simulink model "GravSimple"  (R2020b)
settings: Solver=VariableStepAuto  StartTime=0.0  StopTime=20  MaxStep=0.001  RelTol=1e-3
values from neighbouring files (symbols this model uses):
  b = 1e4    (= 10000)    [calcGrav.m]
  Fpin0 = 4*k0*tauM0/2/(g*1000)    [calcGrav.m]
  GBr = 39.9    [calcGrav.m]
  K = nc*(EA./Ds)    [calcGrav.m]
  M1 = alfa*mc + Mmot + Mwin + Msh    (= 57445.7643225)    [calcGrav.m]
  M2 = (1-alfa)*mc + M    (= 50290)    [calcGrav.m]
  rw0 = 0.562/2    (= 0.281)    [calcGrav.m]
  tau_em = 60e-3    (= 0.06)    [calcGrav.m]    (also in main.m)
  tau_m = tau_w/GB.r    [main.m]
  tau_max = tauM0    [calcGrav.m]
  tauM0 = (M + mc)*g/4/k0    [calcGrav.m]
undefined symbols (not defined in the file or in its folder): PID
libraries: cstblocks x1, pid_lib x1
settings Model: Creator=Pawel  LastModifiedBy=Pawel

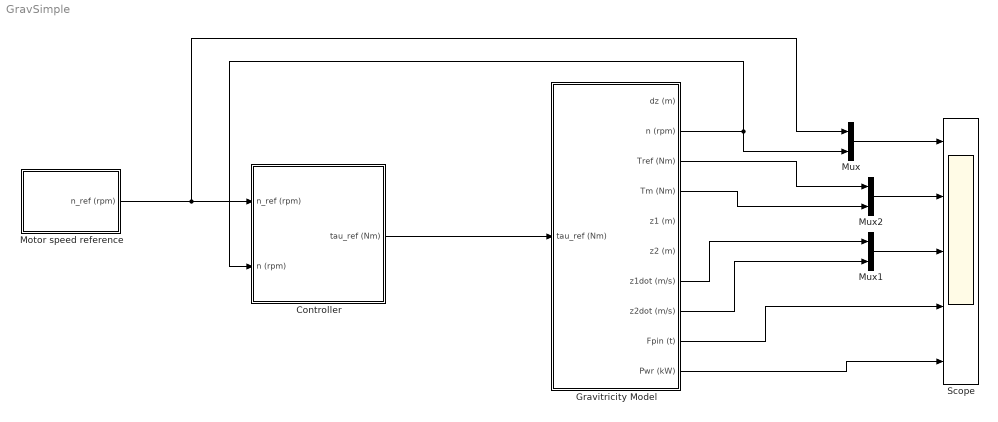
== system GravSimple ==
  Controller : Subsystem
  Gravitricity Model : Subsystem
  Motor speed reference : Subsystem
  Mux : Mux  Inputs=2
  Mux1 : Mux  Inputs=2
  Mux2 : Mux  Inputs=2
  Scope : Scope  NumInputPorts=5
  wires:
  Motor speed reference/1(n_ref (rpm)) -> Mux/1, Controller/1(n_ref (rpm))
  Gravitricity Model/2(n (rpm)) -> Mux/2, Controller/2(n (rpm))
  Controller/1(tau_ref (Nm)) -> Gravitricity Model/1(tau_ref (Nm))
  Mux/1 -> Scope/1
  Gravitricity Model/10(Pwr (kW)) -> Scope/5
  Mux1/1 -> Scope/3
  Gravitricity Model/9(Fpin (t)) -> Scope/4
  Gravitricity Model/7(z1dot (m/s)) -> Mux1/1
  Gravitricity Model/8(z2dot (m/s)) -> Mux1/2
  Mux2/1 -> Scope/2
  Gravitricity Model/3(Tref (Nm)) -> Mux2/1
  Gravitricity Model/4(Tm (Nm)) -> Mux2/2

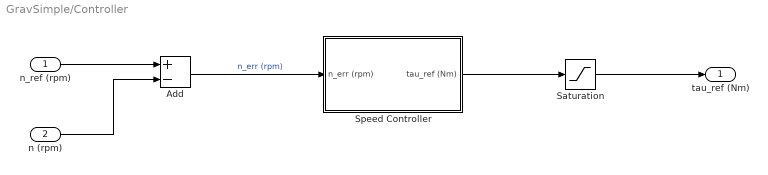
== system GravSimple/Controller ==
  n_ref (rpm) : Inport
  n (rpm) : Inport  Port=2
  Add : Sum  Inputs=+-
  Saturation : Saturate  UpperLimit=tau_max  LowerLimit=-tau_max
  Speed Controller : Subsystem  Variant=on  VariantControlMode=label  LabelModeActiveChoice=Speed_Ctrl_OL
  tau_ref (Nm) : Outport
  wires:
  n_ref (rpm)/1 -> Add/1
  n (rpm)/1 -> Add/2
  Add/1 -> Speed Controller/1(n_err (rpm))  "n_err (rpm)"
  Speed Controller/1(tau_ref (Nm)) -> Saturation/1
  Saturation/1 -> tau_ref (Nm)/1

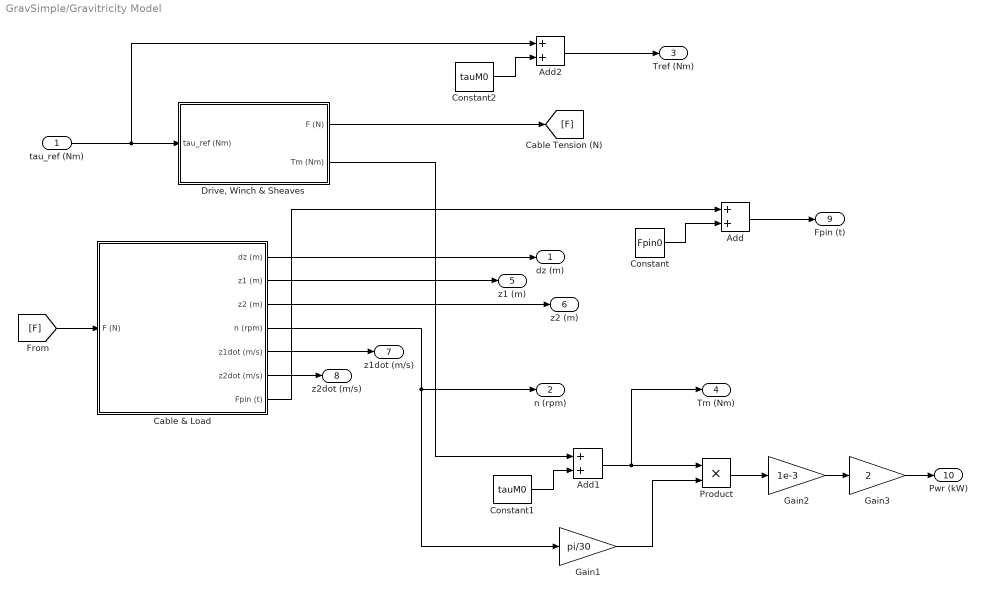
== system GravSimple/Gravitricity Model ==
  tau_ref (Nm) : Inport
  Add : Sum
  Add1 : Sum
  Add2 : Sum
  Cable & Load : Subsystem  Variant=on  VariantControlMode=label  LabelModeActiveChoice=Load_2
  Constant : Constant  Value=Fpin0
  Constant1 : Constant  Value=tauM0
  Constant2 : Constant  Value=tauM0
  "Drive, Winch & Sheaves" : Subsystem  Variant=on  VariantControlMode=label  LabelModeActiveChoice=Drive_2
  Gain1 : Gain  Gain=pi/30
  Gain2 : Gain  Gain=1e-3
  Gain3 : Gain  Gain=2
  Product : Product
  dz (m) : Outport
  n (rpm) : Outport  Port=2
  Tref (Nm) : Outport  Port=3
  Tm (Nm) : Outport  Port=4
  z1 (m) : Outport  Port=5
  z2 (m) : Outport  Port=6
  z1dot (m/s) : Outport  Port=7
  z2dot (m/s) : Outport  Port=8
  Fpin (t) : Outport  Port=9
  Pwr (kW) : Outport  Port=10
  wires:
  tau_ref (Nm)/1 -> Add2/1, "Drive, Winch & Sheaves"/1(tau_ref (Nm))
  "Drive, Winch & Sheaves"/1(F (N)) -> [F]
  [F] -> Cable & Load/1(F (N))
  Cable & Load/1(dz (m)) -> dz (m)/1
  Cable & Load/2(z1 (m)) -> z1 (m)/1
  Cable & Load/3(z2 (m)) -> z2 (m)/1
  Cable & Load/4(n (rpm)) -> Gain1/1, n (rpm)/1
  "Drive, Winch & Sheaves"/2(Tm (Nm)) -> Add1/1
  Cable & Load/7(Fpin (t)) -> Add/1
  Add/1 -> Fpin (t)/1
  Constant/1 -> Add/2
  Constant1/1 -> Add1/2
  Add1/1 -> Tm (Nm)/1, Product/1
  Gain1/1 -> Product/2
  Product/1 -> Gain2/1
  Gain2/1 -> Gain3/1
  Constant2/1 -> Add2/2
  Add2/1 -> Tref (Nm)/1
  Cable & Load/5(z1dot (m/s)) -> z1dot (m/s)/1
  Cable & Load/6(z2dot (m/s)) -> z2dot (m/s)/1
  Gain3/1 -> Pwr (kW)/1

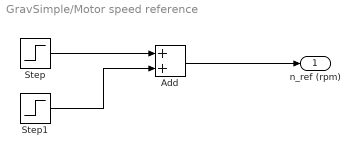
== system GravSimple/Motor speed reference ==
  Add : Sum
  Step : Step  After=1000  SampleTime=0
  Step1 : Step  Time=10  After=-1000  SampleTime=0
  n_ref (rpm) : Outport
  wires:
  Step/1 -> Add/1
  Step1/1 -> Add/2
  Add/1 -> n_ref (rpm)/1

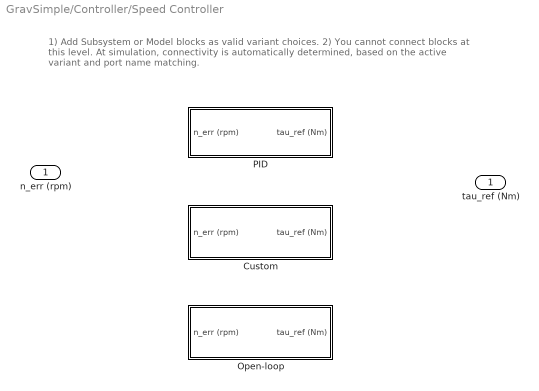
== system GravSimple/Controller/Speed Controller ==
  note: 1) Add Subsystem or Model blocks as valid variant choices.
      | 2) You cannot connect blocks at this level. At simulation, connectivity is automatically
      | determined, based on the active variant and port name matching.
  n_err (rpm) : Inport
  Custom : Subsystem  VariantControl=Speed_Ctrl_Custom
  Open-loop : Subsystem  VariantControl=Speed_Ctrl_OL
  PID : Subsystem  VariantControl=Speed_Ctrl_PID
  tau_ref (Nm) : Outport

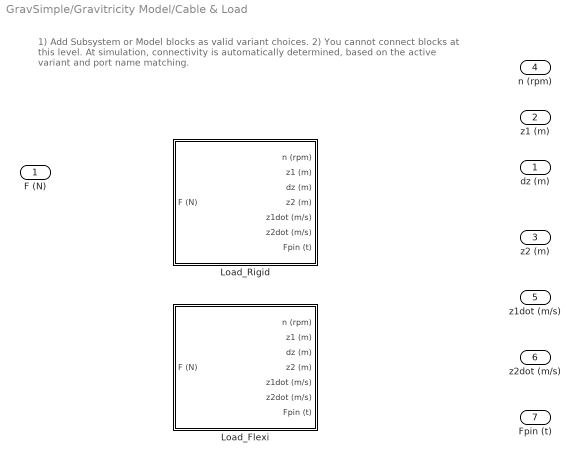
== system GravSimple/Gravitricity Model/Cable & Load ==
  note: 1) Add Subsystem or Model blocks as valid variant choices.
      | 2) You cannot connect blocks at this level. At simulation, connectivity is automatically
      | determined, based on the active variant and port name matching.
  F (N) : Inport
  Load_Flexi : Subsystem  VariantControl=Load_2
  Load_Rigid : Subsystem  VariantControl=Load_1
  dz (m) : Outport
  z1 (m) : Outport  Port=2
  z2 (m) : Outport  Port=3
  n (rpm) : Outport  Port=4
  z1dot (m/s) : Outport  Port=5
  z2dot (m/s) : Outport  Port=6
  Fpin (t) : Outport  Port=7

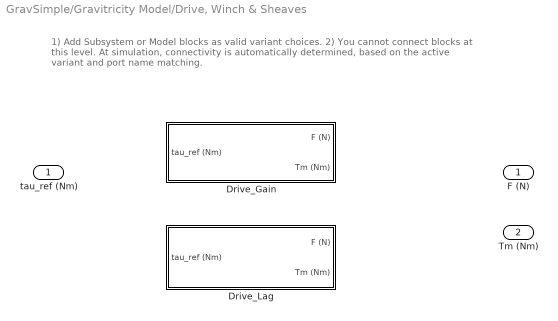
== system GravSimple/Gravitricity Model/Drive, Winch & Sheaves ==
  note: 1) Add Subsystem or Model blocks as valid variant choices.
      | 2) You cannot connect blocks at this level. At simulation, connectivity is automatically
      | determined, based on the active variant and port name matching.
  tau_ref (Nm) : Inport
  Drive_Gain : Subsystem  VariantControl=Drive_1
  Drive_Lag : Subsystem  VariantControl=Drive_2
  F (N) : Outport
  Tm (Nm) : Outport  Port=2

== system GravSimple/Controller/Speed Controller/Custom ==
  n_err (rpm) : Inport
  LTI System : cstblocks/LTI System  sys=sysC  IC=[]
  tau_ref (Nm) : Outport
  wires:
  n_err (rpm)/1 -> LTI System/1
  LTI System/1 -> tau_ref (Nm)/1

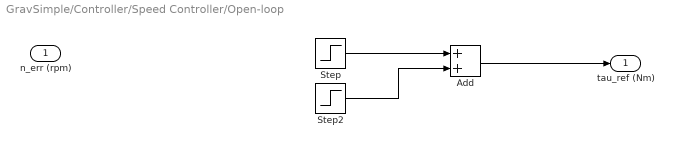
== system GravSimple/Controller/Speed Controller/Open-loop ==
  n_err (rpm) : Inport
  Add : Sum
  Step : Step  Time=5  After=0.5*tau_m  SampleTime=0
  Step2 : Step  Time=5.2  After=-0.5*tau_m  SampleTime=0
  tau_ref (Nm) : Outport
  wires:
  Add/1 -> tau_ref (Nm)/1
  Step/1 -> Add/1
  Step2/1 -> Add/2

== system GravSimple/Controller/Speed Controller/PID ==
  n_err (rpm) : Inport
  PID Controller : pid_lib/PID Controller  Controller=PID  Form=Parallel  TimeDomain=Continuous-time  UseExternalTs=off  SampleTime=-1  IntegratorMethod=Forward Euler  FilterMethod=Forward Euler  ControllerParametersSource=internal  P=PID.P  I=PID.I  D=PID.D  UseFilter=on  N=100  TunerSelectOption=Transfer Function Based (PID Tuner App)  InitialConditionSource=internal  InitialConditionForIntegrator=0  InitialConditionForFilter=0  DifferentiatorICPrevScaledInput=0  ExternalReset=none  TrackingMode=off  Kt=1  LimitOutput=off  SatLimitsSource=internal  UpperSaturationLimit=inf  LowerSaturationLimit=-inf  LinearizeAsGain=on  AntiWindupMode=none  Kb=1  POutMin=[]  POutMax=[]  IOutMin=[]  IOutMax=[]  DOutMin=[]  DOutMax=[]  NOutMin=[]  NOutMax=[]  SumOutMin=[]  SumOutMax=[]  SaturationOutMin=[]  SaturationOutMax=[]  PParamMin=[]  PParamMax=[]  IParamMin=[]  IParamMax=[]  DParamMin=[]  DParamMax=[]  NParamMin=[]  NParamMax=[]  KbParamMin=[]  KbParamMax=[]  KtParamMin=[]  KtParamMax=[]  KbOutMin=[]  KbOutMax=[]  KtOutMin=[]  KtOutMax=[]  IntegratorOutMin=[]  IntegratorOutMax=[]  FilterOutMin=[]  FilterOutMax=[]  SumI1OutMin=[]  SumI1OutMax=[]  SumI2OutMin=[]  SumI2OutMax=[]  SumI3OutMin=[]  SumI3OutMax=[]  SumI4OutMin=[]  SumI4OutMax=[]  SumDOutMin=[]  SumDOutMax=[]  DifferentiatorOutMin=[]  DifferentiatorOutMax=[]  FilterDiffOutCoefMin=[]  FilterDiffOutCoefMax=[]  ReciprocalOutMin=[]  ReciprocalOutMax=[]  SumDenOutMin=[]  SumDenOutMax=[]  SumNumOutMin=[]  SumNumOutMax=[]  DivideOutMin=[]  DivideOutMax=[]  UdiffTsProdOutMin=[]  UdiffTsProdOutMax=[]  NTsProdOutMin=[]  NTsProdOutMax=[]  UintegralTsProdOutMin=[]  UintegralTsProdOutMax=[]  UngainTsProdOutMin=[]  UngainTsProdOutMax=[]  IntegratorContinuousStateAttributes=''  IntegratorStateMustResolveToSignalObject=off  IntegratorRTWStateStorageClass=Auto  FilterContinuousStateAttributes=''  FilterStateMustResolveToSignalObject=off  FilterRTWStateStorageClass=Auto  ParallelPVariant=InternalParameters  IdealPVariant=Disabled  IVariant=InternalParameters  DVariant=InternalParameters  IntegratorVariant=Continuous  SatVariant=Disabled  AWVariant=Passthrough  PCopyVariant=Disabled  TRVariant=Disabled  FdbkBlocksVariant=Forward  IdealPFdbkVariant=Disabled  SatFdbkVariant=Disabled  DerivativeFilterVariant=ContFilter  NVariant=InternalParameters  NCopyVariant=Disabled  FilterICVariant=InternalICsFilter  IntegratorICVariant=InternalICs  ExternalResetVariant=Disabled  TRSumVariant=Passthrough  SumFdbkVariant=Disabled  SumVariant=Sum_PID  TsampFilterVariant=InternalTs  TsampNgainVariant=Passthrough  TsampIntegralVariant=Passthrough  ExternalSaturationOutDataTypeStr=Inherit: Same as second input
  tau_ref (Nm) : Outport
  wires:
  n_err (rpm)/1 -> PID Controller/1
  PID Controller/1 -> tau_ref (Nm)/1

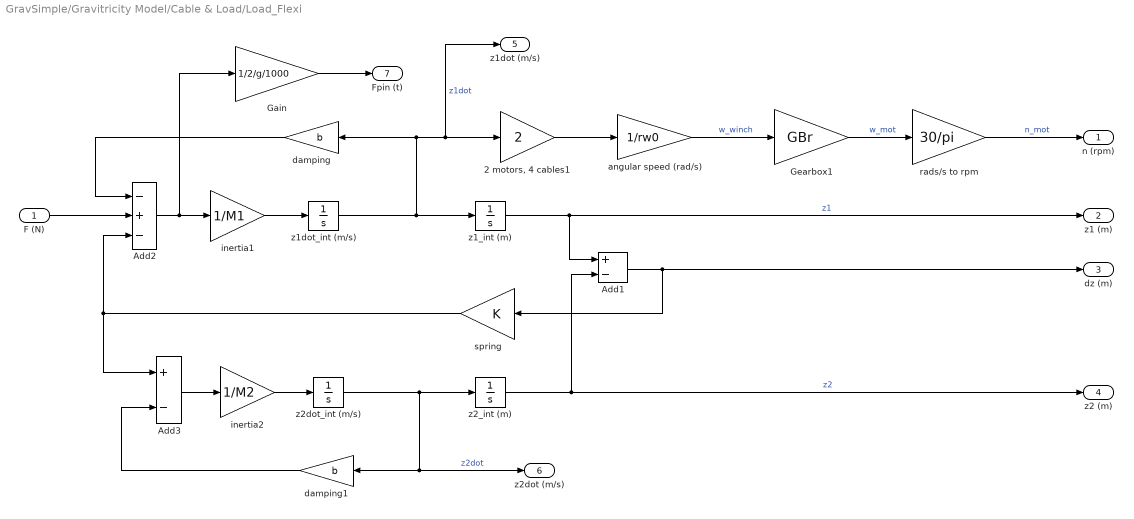
== system GravSimple/Gravitricity Model/Cable & Load/Load_Flexi ==
  F (N) : Inport
  "2 motors, 4 cables1" : Gain  Gain=2
  Add1 : Sum  Inputs=+-
  Add2 : Sum  Inputs=-+-
  Add3 : Sum  Inputs=+-
  Gain : Gain  Gain=1/2/g/1000
  Gearbox1 : Gain  Gain=GBr
  angular speed (rad/s) : Gain  Gain=1/rw0
  damping : Gain  Gain=b
  damping1 : Gain  Gain=b
  inertia1 : Gain  Gain=1/M1
  inertia2 : Gain  Gain=1/M2
  rads/s to rpm : Gain  Gain=30/pi
  spring : Gain  Gain=K
  z1_int (m) : Integrator
  z1dot_int (m/s) : Integrator
  z2_int (m) : Integrator
  z2dot_int (m/s) : Integrator
  n (rpm) : Outport
  z1 (m) : Outport  Port=2
  dz (m) : Outport  Port=3
  z2 (m) : Outport  Port=4
  z1dot (m/s) : Outport  Port=5
  z2dot (m/s) : Outport  Port=6
  Fpin (t) : Outport  Port=7
  wires:
  F (N)/1 -> Add2/2
  inertia2/1 -> z2dot_int (m/s)/1
  Add2/1 -> Gain/1, inertia1/1
  z2_int (m)/1 -> Add1/2, z2 (m)/1  "z2"
  Gearbox1/1 -> rads/s to rpm/1  "w_mot"
  angular speed (rad/s)/1 -> Gearbox1/1  "w_winch"
  z2dot_int (m/s)/1 -> z2_int (m)/1, z2dot (m/s)/1, damping1/1  "z2dot"
  inertia1/1 -> z1dot_int (m/s)/1
  z1_int (m)/1 -> Add1/1, z1 (m)/1  "z1"
  damping1/1 -> Add3/2
  Add3/1 -> inertia2/1
  z1dot_int (m/s)/1 -> z1_int (m)/1, damping/1, z1dot (m/s)/1, "2 motors, 4 cables1"/1  "z1dot"
  Add1/1 -> spring/1, dz (m)/1
  "2 motors, 4 cables1"/1 -> angular speed (rad/s)/1
  spring/1 -> Add2/3, Add3/1
  damping/1 -> Add2/1
  rads/s to rpm/1 -> n (rpm)/1  "n_mot"
  Gain/1 -> Fpin (t)/1

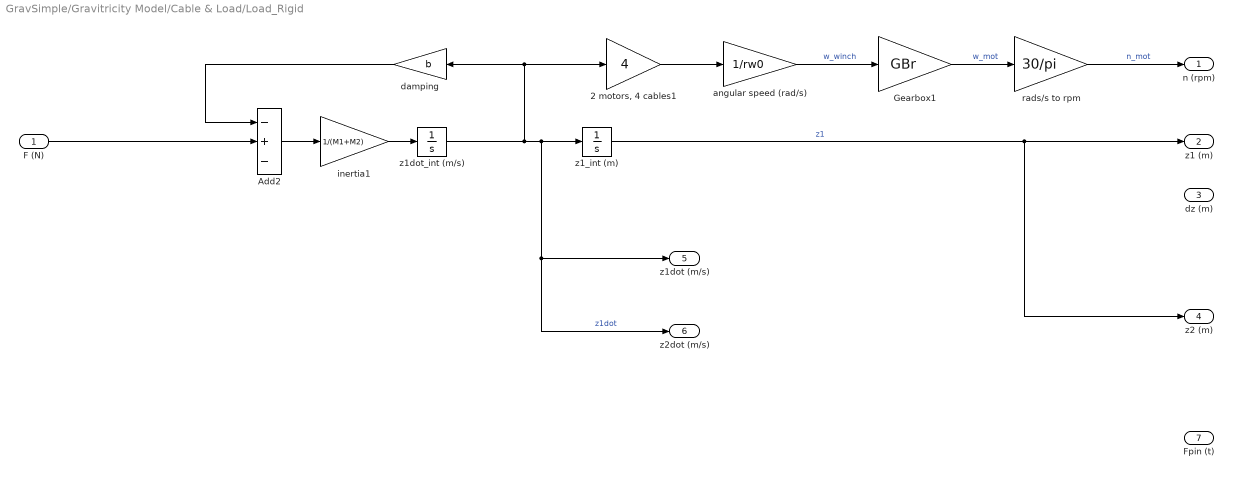
== system GravSimple/Gravitricity Model/Cable & Load/Load_Rigid ==
  F (N) : Inport
  "2 motors, 4 cables1" : Gain  Gain=4
  Add2 : Sum  Inputs=-+-
  Gearbox1 : Gain  Gain=GBr
  angular speed (rad/s) : Gain  Gain=1/rw0
  damping : Gain  Gain=b
  inertia1 : Gain  Gain=1/(M1+M2)
  rads/s to rpm : Gain  Gain=30/pi
  z1_int (m) : Integrator
  z1dot_int (m/s) : Integrator
  n (rpm) : Outport
  z1 (m) : Outport  Port=2
  dz (m) : Outport  Port=3
  z2 (m) : Outport  Port=4
  z1dot (m/s) : Outport  Port=5
  z2dot (m/s) : Outport  Port=6
  Fpin (t) : Outport  Port=7
  wires:
  rads/s to rpm/1 -> n (rpm)/1  "n_mot"
  damping/1 -> Add2/1
  "2 motors, 4 cables1"/1 -> angular speed (rad/s)/1
  z1dot_int (m/s)/1 -> "2 motors, 4 cables1"/1, damping/1, z1dot (m/s)/1, z2dot (m/s)/1, z1_int (m)/1  "z1dot"
  z1_int (m)/1 -> z2 (m)/1, z1 (m)/1  "z1"
  inertia1/1 -> z1dot_int (m/s)/1
  angular speed (rad/s)/1 -> Gearbox1/1  "w_winch"
  Gearbox1/1 -> rads/s to rpm/1  "w_mot"
  Add2/1 -> inertia1/1
  F (N)/1 -> Add2/2

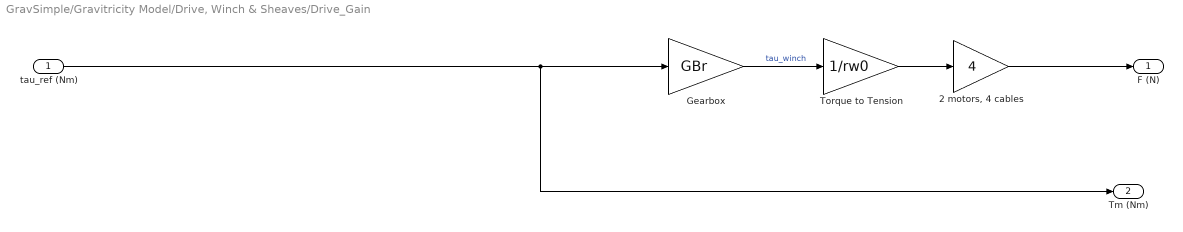
== system GravSimple/Gravitricity Model/Drive, Winch & Sheaves/Drive_Gain ==
  tau_ref (Nm) : Inport
  "2 motors, 4 cables" : Gain  Gain=4
  Gearbox : Gain  Gain=GBr
  Torque to Tension : Gain  Gain=1/rw0
  F (N) : Outport
  Tm (Nm) : Outport  Port=2
  wires:
  Torque to Tension/1 -> "2 motors, 4 cables"/1
  "2 motors, 4 cables"/1 -> F (N)/1
  Gearbox/1 -> Torque to Tension/1  "tau_winch"
  tau_ref (Nm)/1 -> Tm (Nm)/1, Gearbox/1

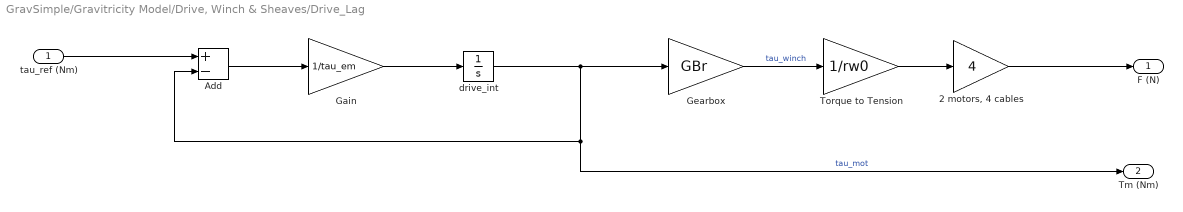
== system GravSimple/Gravitricity Model/Drive, Winch & Sheaves/Drive_Lag ==
  tau_ref (Nm) : Inport
  "2 motors, 4 cables" : Gain  Gain=4
  Add : Sum  Inputs=+-
  Gain : Gain  Gain=1/tau_em
  Gearbox : Gain  Gain=GBr
  Torque to Tension : Gain  Gain=1/rw0
  drive_int : Integrator
  F (N) : Outport
  Tm (Nm) : Outport  Port=2
  wires:
  Gearbox/1 -> Torque to Tension/1  "tau_winch"
  "2 motors, 4 cables"/1 -> F (N)/1
  Gain/1 -> drive_int/1
  Torque to Tension/1 -> "2 motors, 4 cables"/1
  Add/1 -> Gain/1
  drive_int/1 -> Tm (Nm)/1, Add/2, Gearbox/1  "tau_mot"
  tau_ref (Nm)/1 -> Add/1
